simulink library "uavsimBlockset_ElectricPropulsion"  (Simulink 8.8)
settings: Solver=ode45  StartTime=0.0  StopTime=10.0  RelTol=1e-3  EnableMultiTasking=on
undefined symbols (not defined in the file): uavsim
settings Model: Creator=mstolle  LastModifiedBy=j.bolting

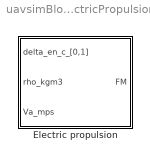
== system uavsimBlockset_ElectricPropulsion ==
  Electric propulsion : Subsystem  mask{mask_C_prop=uavsim.cularis.C_prop, mask_S_prop=uavsim.cularis.S_prop, mask_k_motor=uavsim.cularis.k_motor}
      mask prompts: mask_C_prop "Propeller efficiency constant"; mask_S_prop "Propeller area"; mask_k_motor "Engine constant"

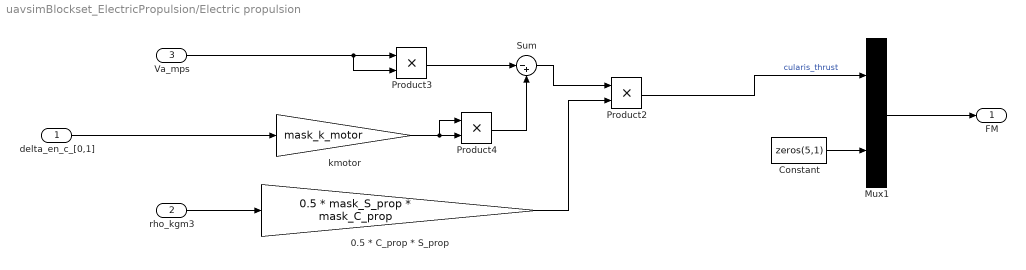
== system uavsimBlockset_ElectricPropulsion/Electric propulsion ==
  delta_en_c_[0,1] : Inport
  rho_kgm3 : Inport  Port=2
  Va_mps : Inport  Port=3
  0.5 * C_prop * S_prop : Gain  Gain=0.5 * mask_S_prop * mask_C_prop
  Constant : Constant  Value=zeros(5,1)
  Mux1 : Mux  Inputs=2
  Product2 : Product  RndMeth=Zero
  Product3 : Product  RndMeth=Zero
  Product4 : Product  RndMeth=Zero
  Sum : Sum  Inputs=|-+
  kmotor : Gain  Gain=mask_k_motor
  FM : Outport
  wires:
  Product2/1 -> Mux1/1  "cularis_thrust"
  Mux1/1 -> FM/1
  Constant/1 -> Mux1/2
  Sum/1 -> Product2/1
  Product3/1 -> Sum/1
  0.5 * C_prop * S_prop/1 -> Product2/2
  kmotor/1 -> Product4/1, Product4/2
  Product4/1 -> Sum/2
  Va_mps/1 -> Product3/2, Product3/1
  rho_kgm3/1 -> 0.5 * C_prop * S_prop/1
  delta_en_c_[0,1]/1 -> kmotor/1
